simulink model "WaterRunner"  (Simulink 7.9)
settings: Solver=ode45  StartTime=0.0  StopTime=10  MaxStep=1e-2  RelTol=1e-3  AbsTol=1e-3
values from neighbouring files (symbols this model uses):
  L1_inertia = 1/12*L1_m*L1_l^2    (= 0.00015759375)    [simParams.m]
  L1_m = 0.5    [simParams.m]
  L2_inertia = 1/12*L2_m*ll_l2^2    (= 3.96033333333e-06)    [simParams.m]
  L2_m = 0.1    [simParams.m]
  l3_angle_0 = u(end-1)    [Foot.m]    (also in calcAngle.m; simParams.m = atan2(ll_l4-YY,XX-ll_Body))
  L3_inertia = 1/12*L2_m*ll_l2^2    (= 3.96033333333e-06)    [simParams.m]
  L3_m = 0.1    [simParams.m]
  L4_inertia = 1/12*L4_m*ll_l4^2    (= 1.8252e-05)    [simParams.m]
  L4_m = 0.1    [simParams.m]
  water_level = u(end)    [Foot.m]    (also in simParams.m = -0.03)
libraries: mblibv1 x19, simulink x1
settings Model: Creator=fumiyaiida  LastModifiedBy=nitisht
settings SolverCC: ZeroCrossControl=DisableAll
settings OptimizationCC: InlineInvariantSignals=on  InitFltsAndDblsToZero=on
settings DebuggingCC: SaveWithParameterizedLinksMsg=none  SignalResolutionControl=TryResolveAllWithWarning  MultiTaskDSMMsg=warning  MultiTaskCondExecSysMsg=none  FcnCallInpInsideContextMsg=Use local settings  StrictBusMsg=None
settings RTWCC: IncludeERTFirstTime=on
settings GRTTargetCC: TargetFcnLib=ansi_tfl_tmw.mat  CombineOutputUpdateFcns=off  GRTInterface=on
settings SimMechanicsCC: WarnOnSingularInitialAssembly=on  VisOnUpdateDiagram=on  VisDuringSimulation=on  VisSampleTime=0.05  AnimationDelay=1  AutoFitVis=GROWTOFIT  LastVizWinPosition=[668 530 1252 448]  CamPosition=[1.38778e-17;0.00693669;11.3889;]  CamTarget=[1.38778e-17;0.00693669;0;]  CamUpVector=[0;1;0;]  CamHeight=0.51  VisBackgroundColor=[0.9;0.9;0.95;]  DefaultBodyColor=[1;0;0;]
settings ConfigurationSet: Description=SimMechanics 2G

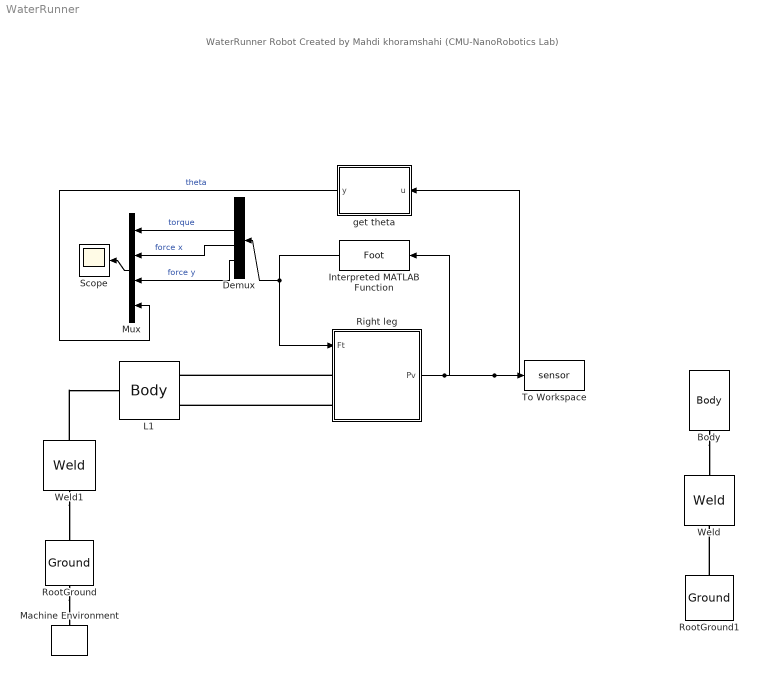
== system WaterRunner ==
  note: WaterRunner Robot
      | Created by Mahdi khoramshahi
      | (CMU-NanoRobotics Lab)
  Body : mblibv1/Bodies/Body  LConnTagsString=CG  UpdateFromCAD=off  DialogClass=MechanicalBodyBlock  Mass=1  MassUnits=kg  InertiaUnits=kg*m^2  Inertia=eye(3)  Shape=Cylinder  ShapeDims=[1 1]  ShapeUnits=m  ShapeUse=false  Density=1  DensityUnits=kg/m^3  DensityUse=false  GraphicsMode=CONVHULL  BodyColorSelMode=COLORPALETTE  BodyColor=[0.83137 0.81569 0.78431]  AttachedToCS=CG  CG=Left$CG$[0 0 0]$Adjoining$Adjoining$m$[0 0 0]$Euler X-Y-Z$deg$WORLD$true$none  WorkingFrames=Left$CS1$[-0.25 0 0]$CG$CG$m$[0 0 0]$Euler X-Y-Z$deg$WORLD$false$none#Left$CS2$[0.25 0 0]$CG$CG$m$[0 0 0]$Euler X-Y-Z$deg$WORLD$false$none  CGPos=[0 0 0]  CGRot=[0 0 0]  CS0Pos=[]  CS0Rot=[]  CS1Pos=[-0.25 0 0]  CS1Rot=[0 0 0]  CS2Pos=[0.25 0 0]  CS2Rot=[0 0 0]  CS3Pos=[]  CS3Rot=[]  CS4Pos=[]  CS4Rot=[]  CS5Pos=[]  CS5Rot=[]  CS6Pos=[]  CS6Rot=[]  CS7Pos=[]  CS7Rot=[]  CS8Pos=[]  CS8Rot=[]  CS9Pos=[]  CS9Rot=[]  CS10Pos=[]  CS10Rot=[]  CS11Pos=[]  CS11Rot=[]  CS12Pos=[]  CS12Rot=[]  CS13Pos=[]  CS13Rot=[]  CS14Pos=[]  CS14Rot=[]  CS15Pos=[]  CS15Rot=[]  CS16Pos=[]  CS16Rot=[]  CS17Pos=[]  CS17Rot=[]  CS18Pos=[]  CS18Rot=[]  CS19Pos=[]  CS19Rot=[]  CS20Pos=[]  CS20Rot=[]
  Demux : Demux  Outputs=6
  Interpreted MATLAB Function : MATLABFcn  MATLABFcn=Foot
  L1 : mblibv1/Bodies/Body  LConnTagsString=CS1  RConnTagsString=CS2|CS3  UpdateFromCAD=on  DialogClass=MechanicalBodyBlock  Mass=L1_m  MassUnits=kg  InertiaUnits=kg*m^2  Inertia=L1_inertia*eye(3)  Shape=Cylinder  ShapeDims=[1 1]  ShapeUnits=m  ShapeUse=false  Density=1  DensityUnits=kg/m^3  DensityUse=false  GraphicsMode=CONVHULL  GraphicsFileName=fourbar-base-1.STL  BodyColorSelMode=COLORPALETTE  BodyColor=[0 0 0]  AttachedToCS=CS1  CG=Right$CG$L1_CG$WORLD$WORLD$m$[0 0 0]$Euler X-Y-Z$deg$WORLD$false$none  WorkingFrames=Left$CS1$L1_CS1$WORLD$WORLD$m$[0 0 0]$Euler X-Y-Z$deg$WORLD$true$none#Right$CS2$L1_CS2$WORLD$WORLD$m$[0 0 0]$Euler X-Y-Z$deg$WORLD$true$none#Right$CS3$L1_CS3$WORLD$WORLD$m$[0 0 0]$Euler X-Y-Z$deg$WORLD$true$none#Right$CS4$L1_CS2$WORLD$WORLD$m$[0 0 0]$Euler X-Y-Z$deg$WORLD$false$none  CGPos=L1_CG  CGRot=[0 0 0]  CS0Pos=[]  CS0Rot=[]  CS1Pos=L1_CS1  CS1Rot=[0 0 0]  CS2Pos=L1_CS2  CS2Rot=[0 0 0]  CS3Pos=L1_CS3  CS3Rot=[0 0 0]  CS4Pos=L1_CS2  CS4Rot=[0 0 0]  CS5Pos=[]  CS5Rot=[]  CS6Pos=[]  CS6Rot=[]  CS7Pos=[]  CS7Rot=[]  CS8Pos=[]  CS8Rot=[]  CS9Pos=[]  CS9Rot=[]  CS10Pos=[]  CS10Rot=[]  CS11Pos=[]  CS11Rot=[]  CS12Pos=[]  CS12Rot=[]  CS13Pos=[]  CS13Rot=[]  CS14Pos=[]  CS14Rot=[]  CS15Pos=[]  CS15Rot=[]  CS16Pos=[]  CS16Rot=[]  CS17Pos=[]  CS17Rot=[]  CS18Pos=[]  CS18Rot=[]  CS19Pos=[]  CS19Rot=[]  CS20Pos=[]  CS20Rot=[]
  Machine Environment : mblibv1/Bodies/Machine Environment  PortType=env  PhysicalDomain=Mechanical  DialogTemplateClass=MECH.MachineEnvironment  SyncWhenCopied=off  Gravity=[0 -9.81 0]  GravityUnits=m/s^2  GravityAsSignal=off  Dimensionality=Auto-detect  AnalysisType=Forward dynamics  LinearAssemblyTolerance=1e-3  LinearAssemblyToleranceUnits=m  AngularAssemblyTolerance=1e-3  AngularAssemblyToleranceUnits=rad  ConstraintSolverType=Stabilizing  ConstraintRelTolerance=1e-4  ConstraintAbsTolerance=1e-4  UseRobustSingularityHandling=off  RedundancyAnalysisToleranceType=Automatically select tolerance  RedundancyAnalysisTolerance=1e-14  StatePerturbationType=Fixed  PerturbationSize=1e-5  VisualizeMachine=on  BodyVisualizationType=Use model default body geometries  BodyColorSelMode=Use model default  DefaultBodyColor=[1 0 0]
  Mux : Mux
  Right leg : Subsystem
  RootGround : mblibv1/Bodies/Ground  UpdateFromCAD=on  LeftPortType=env  RightPortType=workingframe  PhysicalDomain=Mechanical  DialogClass=GroundBlock  CoordPosition=[0 0 0]  CoordPositionUnits=m  StateVectorMgrId=1  MachineId=[1 1]  ShowEnvPort=on
  RootGround1 : mblibv1/Bodies/Ground  UpdateFromCAD=on  LeftPortType=env  RightPortType=workingframe  PhysicalDomain=Mechanical  DialogClass=GroundBlock  CoordPosition=[0 water_level 0]  CoordPositionUnits=m  StateVectorMgrId=0  MachineId=[1 0]  ShowEnvPort=off
  Scope : Scope
      settings: ShowLegends=on  TimeRange=0.4999574105621807  YMin=-1  YMax=1.5
  To Workspace : ToWorkspace  VariableName=sensor  SampleTime=-1  SaveFormat=Structure With Time
  Weld : mblibv1/Joints/Weld  LConnTagsString=__newl0  RConnTagsString=__newr0  UpdateFromCAD=off  NumSAPorts=0  CutJoint=off  MarkAsCut=off  Primitives=weld  PrimitiveProps=W$WORLD$[0 0 0]$weld  DialogClass=JointBlock  WAxis=[0 0 0]
  Weld1 : mblibv1/Joints/Weld  LConnTagsString=__newl0  RConnTagsString=__newr0  UpdateFromCAD=off  NumSAPorts=0  CutJoint=off  MarkAsCut=off  Primitives=weld  PrimitiveProps=W$World$[0 0 0]$weld  DialogClass=JointBlock  WAxis=[0 0 0]
  get theta : MATLAB Function  TreatAsAtomicUnit=on
  wires:
  Right leg/1(Pv) -> Interpreted MATLAB Function/1, To Workspace/1, get theta/1(u)
  Interpreted MATLAB Function/1 -> Right leg/1(Ft), Demux/1
  Mux/1 -> Scope/1
  Demux/3 -> Mux/1  "torque"
  Demux/4 -> Mux/2  "force x"
  Demux/5 -> Mux/3  "force y"
  get theta/1(y) -> Mux/4  "theta"
  connections:
  RootGround/LConn1 -- Machine Environment/RConn1
  RootGround1/RConn1 -- Weld/LConn1
  Body/LConn1 -- Weld/RConn1
  Weld1/LConn1 -- RootGround/RConn1
  Weld1/RConn1 -- L1/LConn1
  Right leg/LConn1 -- L1/RConn1
  Right leg/LConn2 -- L1/RConn2

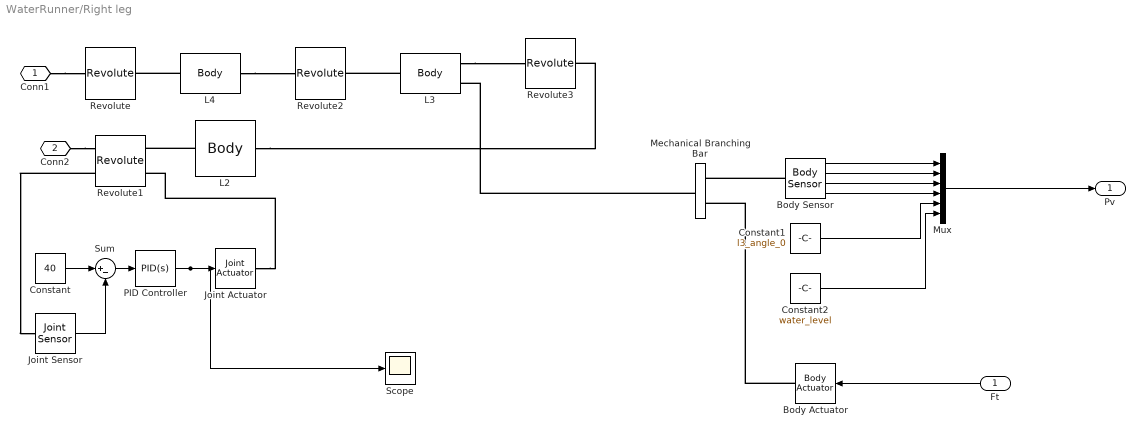
== system WaterRunner/Right leg ==
  Ft : Inport
  Body Actuator : mblibv1/Sensors &  Actuators/Body Actuator  UpdateFromCAD=off  PhysicalDomain=Mechanical  PortType=blob  ActuationStyle=Force  AngleUnits=deg  ArcVelocityUnits=deg/s  ArcAccelerationUnits=deg/s^2  CoordPositionUnits=m  VelocityUnits=m/s  AccelerationUnits=m/s^2  ForceUnits=N  TorqueUnits=N*m  ActiveIO=on  Width=6  DialogClass=MechanicalActuatorBlock  ReferenceFrame=Absolute (World)  Angle=off  CoordPosition=on  Force=on  Torque=on
  Body Sensor : mblibv1/Sensors &  Actuators/Body Sensor  UpdateFromCAD=off  PhysicalDomain=Mechanical  PortType=blob  Muxed=off  Pose=on  Angle=on  AngleUnits=deg  ArcVelocity=on  ArcVelocityUnits=rad/s  ArcAcceleration=off  ArcAccelerationUnits=deg/s^2  CoordPosition=on  CoordPositionUnits=m  Velocity=on  VelocityUnits=m/s  Acceleration=off  AccelerationUnits=m/s^2  Quaternion=on  QuaternionDT=off  QuaternionDDT=off  QuaternionUnits=off  OutputVector=[1]  ActiveIO=on  Width=18  DialogClass=MechanicalSensorBlock  ReferenceFrame=Absolute (World)
  Constant : Constant  Value=40
  Constant1 : Constant  Value=l3_angle_0
  Constant2 : Constant  Value=water_level
  Joint Actuator : mblibv1/Sensors &  Actuators/Joint Actuator  UpdateFromCAD=off  PhysicalDomain=Mechanical  PortType=blob  ActuationStyle=Force  AngleUnits=deg  ArcVelocityUnits=deg/s  ArcAccelerationUnits=deg/s^2  CoordPositionUnits=m  VelocityUnits=m/s  AccelerationUnits=m/s^2  ForceUnits=N  TorqueUnits=N*m  ActiveIO=on  Width=1  DialogClass=MechanicalActuatorBlock  Primitive=R1  ReferenceFrame=Absolute (World)
  Joint Sensor : mblibv1/Sensors &  Actuators/Joint Sensor  UpdateFromCAD=off  PhysicalDomain=Mechanical  PortType=blob  Muxed=on  Pose=off  Angle=off  AngleUnits=deg  ArcVelocity=on  ArcVelocityUnits=rad/s  ArcAcceleration=off  ArcAccelerationUnits=deg/s^2  CoordPosition=on  CoordPositionUnits=m  Velocity=off  VelocityUnits=m/s  Acceleration=off  AccelerationUnits=m/s^2  Quaternion=on  QuaternionDT=off  QuaternionDDT=off  QuaternionUnits=off  OutputVector=[1]  ActiveIO=on  Width=1  DialogClass=MechanicalSensorBlock  Primitive=R1  Force=off  ForceUnits=N  Torque=off  TorqueUnits=N*m  ReferenceFrame=Absolute (World)  ReactionSensedSide=Base  ReactionReferenceFrame=Absolute (World)  ReactionForce=off  ReactionForceUnits=N  ReactionMoment=off  ReactionMomentUnits=N*m
  L2 : mblibv1/Bodies/Body  LConnTagsString=CS2  RConnTagsString=CS1  UpdateFromCAD=on  DialogClass=MechanicalBodyBlock  Mass=L2_m  MassUnits=kg  InertiaUnits=kg*m^2  Inertia=L2_inertia*eye(3)  Shape=Cylinder  ShapeDims=[1 1]  ShapeUnits=m  ShapeUse=false  Density=1  DensityUnits=kg/m^3  DensityUse=false  GraphicsMode=CONVHULL  GraphicsFileName=fourbar-Bar3-1.STL  BodyColorSelMode=COLORPALETTE  BodyColor=[0;0.498039;0]  AttachedToCS=CS1  CG=Right$CG$L2_CG$WORLD$WORLD$m$[0 0 0]$Euler X-Y-Z$deg$WORLD$false$none  WorkingFrames=Right$CS1$L2_CS1$WORLD$WORLD$m$[0 0 0]$Euler X-Y-Z$rad$WORLD$true$none#Left$CS2$L2_CS2$WORLD$WORLD$m$[0 0 0]$Euler X-Y-Z$deg$WORLD$true$none  CGPos=L2_CG  CGRot=[0 0 0]  CS0Pos=[]  CS0Rot=[]  CS1Pos=L2_CS1  CS1Rot=[0 0 0]  CS2Pos=L2_CS2  CS2Rot=[0 0 0]  CS3Pos=[]  CS3Rot=[]  CS4Pos=[]  CS4Rot=[]  CS5Pos=[]  CS5Rot=[]  CS6Pos=[]  CS6Rot=[]  CS7Pos=[]  CS7Rot=[]  CS8Pos=[]  CS8Rot=[]  CS9Pos=[]  CS9Rot=[]  CS10Pos=[]  CS10Rot=[]  CS11Pos=[]  CS11Rot=[]  CS12Pos=[]  CS12Rot=[]  CS13Pos=[]  CS13Rot=[]  CS14Pos=[]  CS14Rot=[]  CS15Pos=[]  CS15Rot=[]  CS16Pos=[]  CS16Rot=[]  CS17Pos=[]  CS17Rot=[]  CS18Pos=[]  CS18Rot=[]  CS19Pos=[]  CS19Rot=[]  CS20Pos=[]  CS20Rot=[]
  L3 : mblibv1/Bodies/Body  LConnTagsString=CS2|CS3  RConnTagsString=CS1  UpdateFromCAD=on  DialogClass=MechanicalBodyBlock  Mass=L3_m  MassUnits=kg  InertiaUnits=kg*m^2  Inertia=L3_inertia*eye(3)  Shape=Cylinder  ShapeDims=[1 1]  ShapeUnits=m  ShapeUse=false  Density=1  DensityUnits=kg/m^3  DensityUse=false  GraphicsMode=CONVHULL  GraphicsFileName=fourbar-Bar2-1.STL  BodyColorSelMode=COLORPALETTE  BodyColor=[0 0 1]  AttachedToCS=CS1  CG=Right$CG$L3_CG$WORLD$WORLD$m$[0 0 0]$Euler X-Y-Z$deg$WORLD$false$none  WorkingFrames=Right$CS1$L3_CS1$WORLD$WORLD$m$[0 0 0]$Euler X-Y-Z$deg$WORLD$true$none#Left$CS2$L3_CS2$WORLD$WORLD$m$[0 0 0]$Euler X-Y-Z$deg$WORLD$true$none#Left$CS3$L3_CS3$WORLD$WORLD$m$[0 0 0]$Euler X-Y-Z$deg$WORLD$true$none  CGPos=L3_CG  CGRot=[0 0 0]  CS0Pos=[]  CS0Rot=[]  CS1Pos=L3_CS1  CS1Rot=[0 0 0]  CS2Pos=L3_CS2  CS2Rot=[0 0 0]  CS3Pos=L3_CS3  CS3Rot=[0 0 0]  CS4Pos=[]  CS4Rot=[]  CS5Pos=[]  CS5Rot=[]  CS6Pos=[]  CS6Rot=[]  CS7Pos=[]  CS7Rot=[]  CS8Pos=[]  CS8Rot=[]  CS9Pos=[]  CS9Rot=[]  CS10Pos=[]  CS10Rot=[]  CS11Pos=[]  CS11Rot=[]  CS12Pos=[]  CS12Rot=[]  CS13Pos=[]  CS13Rot=[]  CS14Pos=[]  CS14Rot=[]  CS15Pos=[]  CS15Rot=[]  CS16Pos=[]  CS16Rot=[]  CS17Pos=[]  CS17Rot=[]  CS18Pos=[]  CS18Rot=[]  CS19Pos=[]  CS19Rot=[]  CS20Pos=[]  CS20Rot=[]
  L4 : mblibv1/Bodies/Body  LConnTagsString=CS2  RConnTagsString=CS1  UpdateFromCAD=on  DialogClass=MechanicalBodyBlock  Mass=L4_m  MassUnits=kg  InertiaUnits=kg*m^2  Inertia=L4_inertia*eye(3)  Shape=Cylinder  ShapeDims=[1 1]  ShapeUnits=m  ShapeUse=false  Density=1  DensityUnits=kg/m^3  DensityUse=false  GraphicsMode=CONVHULL  GraphicsFileName=fourbar-Bar1-1.STL  BodyColorSelMode=COLORPALETTE  BodyColor=[0.847059;0.160784;0]  AttachedToCS=CS1  CG=Right$CG$L4_CG$WORLD$WORLD$m$[0 0 0]$Euler X-Y-Z$deg$WORLD$false$none  WorkingFrames=Right$CS1$L4_CS1$WORLD$WORLD$m$[0 0 0]$Euler X-Y-Z$deg$WORLD$true$none#Left$CS2$L4_CS2$WORLD$WORLD$m$[0 0 0]$Euler X-Y-Z$deg$WORLD$true$none  CGPos=L4_CG  CGRot=[0 0 0]  CS0Pos=[]  CS0Rot=[]  CS1Pos=L4_CS1  CS1Rot=[0 0 0]  CS2Pos=L4_CS2  CS2Rot=[0 0 0]  CS3Pos=[]  CS3Rot=[]  CS4Pos=[]  CS4Rot=[]  CS5Pos=[]  CS5Rot=[]  CS6Pos=[]  CS6Rot=[]  CS7Pos=[]  CS7Rot=[]  CS8Pos=[]  CS8Rot=[]  CS9Pos=[]  CS9Rot=[]  CS10Pos=[]  CS10Rot=[]  CS11Pos=[]  CS11Rot=[]  CS12Pos=[]  CS12Rot=[]  CS13Pos=[]  CS13Rot=[]  CS14Pos=[]  CS14Rot=[]  CS15Pos=[]  CS15Rot=[]  CS16Pos=[]  CS16Rot=[]  CS17Pos=[]  CS17Rot=[]  CS18Pos=[]  CS18Rot=[]  CS19Pos=[]  CS19Rot=[]  CS20Pos=[]  CS20Rot=[]
  Mechanical Branching Bar : mblibv1/Utilities/Mechanical Branching Bar  LConnTagsString=_newl0  RConnTagsString=__newr0|SA2  UpdateFromCAD=off  DialogClass=MechanicalBranchingBarBlock  NumSAPorts=2
  Mux : Mux  Inputs=6
  PID Controller : simulink/Continuous/PID Controller  Controller=PID  TimeDomain=Continuous-time  SampleTime=1  IntegratorMethod=Forward Euler  FilterMethod=Forward Euler  Form=Parallel  P=1  I=1  D=0  N=100  InitialConditionSource=internal  InitialConditionForIntegrator=0  InitialConditionForFilter=0  ExternalReset=none  LimitOutput=off  UpperSaturationLimit=inf  LowerSaturationLimit=-inf  LinearizeAsGain=off  AntiWindupMode=none  Kb=1  TrackingMode=off  Kt=1  PParamMin=[]  PParamMax=[]  IParamMin=[]  IParamMax=[]  DParamMin=[]  DParamMax=[]  NParamMin=[]  NParamMax=[]  KbParamMin=[]  KbParamMax=[]  KtParamMin=[]  KtParamMax=[]  POutMin=[]  POutMax=[]  IOutMin=[]  IOutMax=[]  DOutMin=[]  DOutMax=[]  NOutMin=[]  NOutMax=[]  KbOutMin=[]  KbOutMax=[]  KtOutMin=[]  KtOutMax=[]  IntegratorOutMin=[]  IntegratorOutMax=[]  FilterOutMin=[]  FilterOutMax=[]  SumOutMin=[]  SumOutMax=[]  SumI1OutMin=[]  SumI1OutMax=[]  SumI2OutMin=[]  SumI2OutMax=[]  SumI3OutMin=[]  SumI3OutMax=[]  SumDOutMin=[]  SumDOutMax=[]  SaturationOutMin=[]  SaturationOutMax=[]  IntegratorContinuousStateAttributes=''  IntegratorStateMustResolveToSignalObject=off  IntegratorRTWStateStorageClass=Auto  FilterContinuousStateAttributes=''  FilterStateMustResolveToSignalObject=off  FilterRTWStateStorageClass=Auto
  Revolute : mblibv1/Joints/Revolute  LConnTagsString=__newl0  RConnTagsString=__newr0  UpdateFromCAD=on  NumSAPorts=0  CutJoint=off  MarkAsCut=off  Primitives=prismatic  PrimitiveProps=R1$World$[0,0,1]$revolute  DialogClass=JointBlock  R1Axis=[0,0,1]
  Revolute1 : mblibv1/Joints/Revolute  LConnTagsString=__newl0|SA1  RConnTagsString=__newr0|SA1  UpdateFromCAD=on  NumSAPorts=2  CutJoint=off  MarkAsCut=off  Primitives=prismatic  PrimitiveProps=R1$World$[0,0,1]$revolute  DialogClass=JointBlock  R1Axis=[0,0,1]
  Revolute2 : mblibv1/Joints/Revolute  LConnTagsString=__newl0  RConnTagsString=__newr0  UpdateFromCAD=on  NumSAPorts=0  CutJoint=off  MarkAsCut=off  Primitives=prismatic  PrimitiveProps=R1$World$[0,0,1]$revolute  DialogClass=JointBlock  R1Axis=[0,0,1]
  Revolute3 : mblibv1/Joints/Revolute  LConnTagsString=__newl0  RConnTagsString=__newr0  UpdateFromCAD=on  NumSAPorts=0  CutJoint=on  MarkAsCut=off  Primitives=prismatic  PrimitiveProps=R1$World$[0,0,1]$revolute  DialogClass=JointBlock  R1Axis=[0,0,1]
  Scope : Scope
      settings: YMin=-0.25  YMax=0.25
  Sum : Sum  Inputs=|+-
  Conn1 : PMIOPort  Port=1  Side=Left
  Conn2 : PMIOPort  Port=2  Side=Left
  Pv : Outport
  wires:
  Sum/1 -> PID Controller/1
  PID Controller/1 -> Joint Actuator/1, Scope/1
  Joint Sensor/1 -> Sum/2
  Constant/1 -> Sum/1
  Mux/1 -> Pv/1
  Constant2/1 -> Mux/6
  Constant1/1 -> Mux/5
  Body Sensor/1 -> Mux/1
  Body Sensor/2 -> Mux/2
  Body Sensor/3 -> Mux/3
  Body Sensor/4 -> Mux/4
  Ft/1 -> Body Actuator/1
  connections:
  Revolute1/LConn2 -- Joint Sensor/LConn1
  L2/LConn1 -- Revolute3/RConn1
  L2/RConn1 -- Revolute1/RConn1
  L3/LConn1 -- Revolute3/LConn1
  L3/RConn1 -- Revolute2/RConn1
  L4/LConn1 -- Revolute2/LConn1
  L4/RConn1 -- Revolute/RConn1
  Conn1/RConn1 -- Revolute/LConn1
  Conn2/RConn1 -- Revolute1/LConn1
  Mechanical Branching Bar/LConn1 -- L3/LConn2
  Body Sensor/LConn1 -- Mechanical Branching Bar/RConn1
  Body Actuator/RConn1 -- Mechanical Branching Bar/RConn2
  Joint Actuator/RConn1 -- Revolute1/RConn2

== matlab function get theta ==
  data: u input double; y output double
function y = fcn(u)
%#codegen

 % u = [x y z   x' y' z' Rx'  Ry'  Rz' rot1 ... rot9    angle0 water_level]
    % ind  1 2 3   4  5  6   7   8     9   10       18     19      20

    %Read in variables
    l3_angle_0 = u(end-1);
    theta = atan2(u(11),u(10))+l3_angle_0;
	y = theta;
end
